simulink model "FOC_Motor_Sensorless"  (R2025b)
settings: Solver=VariableStepAuto  StartTime=0.0  StopTime=8  RelTol=1e-3
undefined symbols (not defined in the file or in its folder): adc, dataRange, encoder, inverter, paramAdcAmperePerCount, paramAdcCalibrationSamples, paramAdcCountAtZeroAmpere, paramAdcEnablecalibration, paramCurrentControlSatVoltage, paramOverCurrentDuration, paramOverCurrentEnable, paramOverCurrentLimit, paramPwmCompareAtZeroVolt, paramPwmCompareMax, paramPwmComparePerVolt, paramVelocityControlSatCurrent, PI_params, pmsm, PU_System, pwm, sampleTime
libraries: fl_lib x12, nesl_utility x12, mcbeeMathTransformLib x5, mcbcontrolslib x5, ee_lib x4, slpidlib x2, simulink x2, mcbhdlpositiondecoderlib x2, mcbplantlib x1, autolibpmsmexterior x1, eeGeneralControl x1, SignalEditorBlockLib x1
(part 2 of 2)

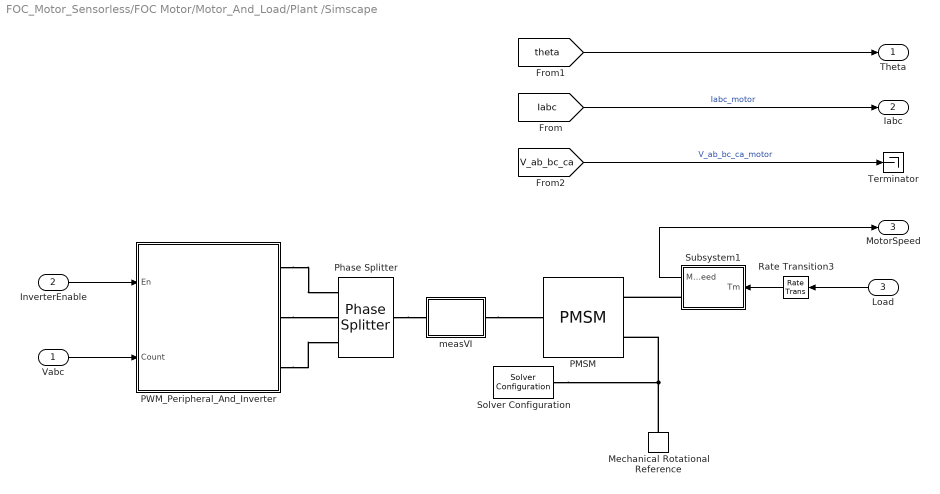
== system FOC_Motor_Sensorless/FOC Motor/Motor_And_Load/Plant /Simscape ==
  Vabc : Inport
  InverterEnable : Inport  Port=2
  Load : Inport  Port=3
  Mechanical Rotational Reference : fl_lib/Mechanical/Rotational Elements/Mechanical Rotational Reference
  PMSM : ee_lib/Electromechanical/Permanent Magnet/PMSM  port_option=ee.enum.threePhasePort.composite  winding_type=ee.enum.statorconnection.wye  machine_param=ee.enum.pmsm.parameterization.constant  nPolePairs=pmsm.p  pmflux_param=ee.enum.pmflux.fluxlinkage  pm_flux_linkage=pmsm.FluxPM Wb  torque_constant=0.18 N*m/A  back_emf_constant=0.18 V/(rad/s)  stator_param=ee.enum.statorparam.LdLqL0  Ld=pmsm.Ld H  Lq=pmsm.Lq H  idVec=[-200, 0, 200] A  iqVec=[-200, 0, 200] A  LdMatrix=0.0002 * ones(3, 3) H  LqMatrix=0.0002 * ones(3, 3) H  PmMatrix=0.1 * ones(3, 3) Wb  ktMatrix=0.18 * ones(3, 3) N*m/A  keMatrix=0.18 * ones(3, 3) V/(rad/s)  L0=0 H  Ls=0.0002 H  Lm=-0.00002 H  Ms=0.00002 H  Rs=pmsm.Rs Ohm  zero_sequence=ee.enum.park.zerosequence.exclude  axes_param=ee.enum.rotorangle.daxis  loss_param=ee.enum.ironloss.none  losses_oc=[0, 0, 0] W  losses_sc=[0, 0, 0] W  f_losses=60 Hz  Isc_losses=95 A  J=pmsm.J kg*m^2  lam=pmsm.B N*m/(rad/s)  i_d_specify=off  i_d_priority=None  i_d=0 A  i_d_nominal_specify=off  i_d_nominal_value=1  i_d_nominal_unit=A  i_q_specify=off  i_q_priority=None  i_q=0 A  i_q_nominal_specify=off  i_q_nominal_value=1  i_q_nominal_unit=A  torque_specify=off  torque_priority=None  torque=0 N*m  torque_nominal_specify=off  torque_nominal_value=1  torque_nominal_unit=N*m  angular_velocity_specify=off  angular_velocity_priority=High  angular_velocity=0 rpm  angular_velocity_nominal_specify=off  angular_velocity_nominal_value=1  angular_velocity_nominal_unit=rpm  angular_position_specify=off  angular_position_priority=High  angular_position=0 deg  angular_position_nominal_specify=off  angular_position_nominal_value=1  angular_position_nominal_unit=deg  alpha=3.93e-3 1/K  alpha_flux=-0.001 1/K  Tmeas=298.15 K  stator_thermal_mass=100 J/K  rotor_thermal_mass=200 J/K  Rm_percent_rotor=90  Rd_percent_rotor=30  temperatureA_specify=off  temperatureA_priority=High  temperatureA=25 degC  temperatureA_nominal_specify=off  temperatureA_nominal_value=1  temperatureA_nominal_unit=degC  temperatureB_specify=off  temperatureB_priority=High  temperatureB=25 degC  temperatureB_nominal_specify=off  temperatureB_nominal_value=1  temperatureB_nominal_unit=degC  temperatureC_specify=off  temperatureC_priority=High  temperatureC=25 degC  temperatureC_nominal_specify=off  temperatureC_nominal_value=1  temperatureC_nominal_unit=degC  temperatureR_specify=off  temperatureR_priority=High  temperatureR=25 degC  temperatureR_nominal_specify=off  temperatureR_nominal_value=1  temperatureR_nominal_unit=degC
      settings: InternalSimscapePortConfiguration="{\"Bottom\":[],\"Left\":[{\"id\":\"N\",\"label\":\"~\",\"type\":\"foundation.electrical.three_phase\"}],\"Right\":[{\"id\":\"R\",\"label\":\"R\",\"type\":\"foundation.mechanical.rotational.rotational\"},{\"id\":\"C\",\"label\":\"C\",\"type\":\"foundation.mechanical.rotational.rotational\"}],\"Top\":[]}"
  PWM_Peripheral_And_Inverter : Subsystem  VariantControl=variantPwm == enumPwm.behavior
      mask Display:
      | image('pwmPeripheralAndInverterMask.png')
      | port_label('input',1,'En')
      | port_label('input',2,'Compare')
      | text(0.98, 0.64, 'A', 'HorizontalAlignment', 'Right')
      | text(0.98, 0.38, 'B', 'HorizontalAlignment', 'Right')
      | text(0.98, 0.12, 'C', 'HorizontalAlignment', 'Right')
  Phase Splitter : ee_lib/Connectors & References/Phase Splitter
  Rate Transition3 : RateTransition  Deterministic=off  OutPortSampleTime=sampleTime.CurrentControl/2
  Solver Configuration : nesl_utility/Solver Configuration  PhysicalDomain=network_engine_domain  SubClassName=solver  LeftPortType=input  RightPortType=generic  Tones=[]  Harmonics=[]  SimulateNoise=off  Profile=off  UseLocalSampling=off  EnableSwitchedLinearOptims=on  FrequencyDomain=off  UseCCode=off  RelTol=0.001  AbsTol=1e-06  MinStep=1e-09  ToWorkspace=off  RevertToSquareIcSolve=off  NumHomotopyIterations=100  PhasorMode=off  PhasorModeNumHarmonics=1  ConsistencySolver=NEWTON_FTOL  IndexReductionMethod=DerivativeReplacement  DoDC=off  ResidualTolerance=1e-09  ConsistencyTolSource=GLOBAL  ConsistencyAbsTol=0.001  ConsistencyRelTol=0.001  ConsistencyTolFactor=0.001  UseLocalSolver=on  LocalSolverChoice=NE_BACKWARD_EULER_ADVANCER  ResolveIndetEquations=on  FunctionEvalNumThread=1  LocalSolverSampleTime=sampleTime.CurrentControl/2  DoFixedCost=on  MaxNonlinIter=3  MaxModeIter=2  ComputeImpulses=off  ImpulseIterations=1  LinearAlgebra=Full  LinearAlgebraNumThread=0  EquationFormulation=NE_TIME_EF  DelaysMemoryBudget=1024  AutomaticFiltering=off  FilteringTimeConstant=0.001  PartitionStorageMethod=AS_NEEDED  PartitionMemoryBudget=1024  PartitionMethod=ROBUST  MultibodyUseLocalSolver=off  MultibodyLocalSolverChoice=ODE1  MultibodyLocalSolverSampleTime=0.001
  Subsystem1 : Subsystem
  Terminator : Terminator
  measVI : Subsystem
  Theta : Outport
  Iabc : Outport  Port=2
  MotorSpeed : Outport  Port=3
  wires:
  Subsystem1/1(MotorSpeed) -> MotorSpeed/1
  [V_ab_bc_ca] -> Terminator/1  "V_ab_bc_ca_motor"
  Rate Transition3/1 -> Subsystem1/1(Tm)
  [theta] -> Theta/1
  [Iabc] -> Iabc/1  "Iabc_motor"
  Load/1 -> Rate Transition3/1
  Vabc/1 -> PWM_Peripheral_And_Inverter/2(Count)
  InverterEnable/1 -> PWM_Peripheral_And_Inverter/1(En)
  connections:
  Subsystem1/RConn1 -- PMSM/RConn1
  Mechanical Rotational Reference/LConn1 -- PMSM/RConn2 -- Solver Configuration/RConn1
  measVI/RConn1 -- PMSM/LConn1
  Phase Splitter/LConn1 -- measVI/LConn1
  PWM_Peripheral_And_Inverter/RConn1 -- Phase Splitter/RConn1
  PWM_Peripheral_And_Inverter/RConn2 -- Phase Splitter/RConn2
  PWM_Peripheral_And_Inverter/RConn3 -- Phase Splitter/RConn3

== system FOC_Motor_Sensorless/FOC Motor/Motor_And_Load/Sensor_Measurements/Get_PU  ==
  rad : Inport
  Constant2 : Constant  Value=2*pi  OutDataTypeStr=single  SampleTime=-1
  Get_PU : Gain  Gain=1/(2*pi)  RndMeth=Simplest  OutDataTypeStr=Inherit: Same as input
  Mod : Math  Operator=mod
  PU : Outport  VectorParamsAs1DForOutWhenUnconnected=off
  wires:
  rad/1 -> Mod/1
  Constant2/1 -> Mod/2
  Mod/1 -> Get_PU/1
  Get_PU/1 -> PU/1

== system FOC_Motor_Sensorless/FOC Motor/Motor_And_Load/Sensor_Measurements/Wrap ==
  in : Inport
  Constant2 : Constant  OutDataTypeStr=single  SampleTime=-1
  Mod : Math  Operator=mod
  out : Outport  VectorParamsAs1DForOutWhenUnconnected=off
  wires:
  in/1 -> Mod/1
  Constant2/1 -> Mod/2
  Mod/1 -> out/1

== system FOC_Motor_Sensorless/FOC Motor/Controller_Algorithm_Local/Algorithm_HDL/FOC_Current_Control/ADC_Count_To_Current ==
  note: ADC Count to Current
  Count : Inport  OutMin=0  OutMax=2^16-1  OutDataTypeStr=uint16  LockScale=on
  ADC_Offsets : Inport  Port=2
  Add : Sum  Inputs=+-  OutDataTypeStr=int16  LockScale=on
  Data_Type_Convert : DataTypeConversion  OutDataTypeStr=int32  SaturateOnIntegerOverflow=off  RndMeth=Floor  LockScale=on
  Product : Product  OutDataTypeStr=fixdt(1,32,19)
  Sat : Saturate  UpperLimit=dataRange.PhaseCurrent.Max  LowerLimit=dataRange.PhaseCurrent.Min  OutDataTypeStr=fixdt(1,16,11)
      settings: AttributesFormatString=-----------------\nLower = %<LowerLimit>\nUpper = %<UpperLimit>
  Scalar : Constant  Value=paramAdcAmperePerCount  OutDataTypeStr=fixdt(1,16,19)  SampleTime=-1
  Current : Outport  VectorParamsAs1DForOutWhenUnconnected=off
  ADC_Counts : Outport  Port=2  VectorParamsAs1DForOutWhenUnconnected=off
  wires:
  ADC_Offsets/1 -> Add/2
  Scalar/1 -> Product/2
  Add/1 -> Product/1
  Count/1 -> ADC_Counts/1, Data_Type_Convert/1
  Data_Type_Convert/1 -> Add/1
  Product/1 -> Sat/1
  Sat/1 -> Current/1

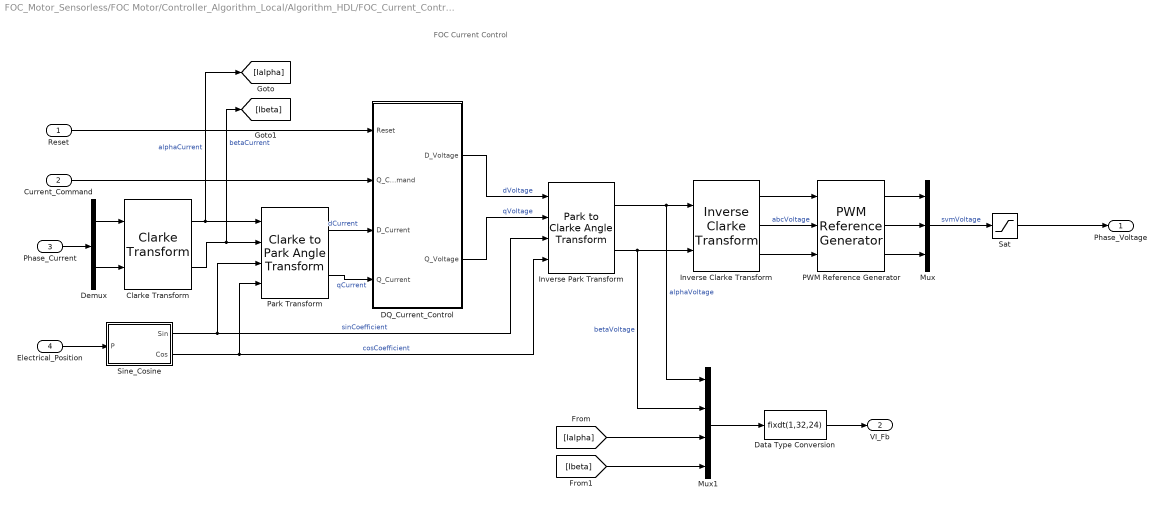
== system FOC_Motor_Sensorless/FOC Motor/Controller_Algorithm_Local/Algorithm_HDL/FOC_Current_Control/FOC_Current_Control ==
  note: FOC Current Control
  Reset : Inport  SampleTime=sampleTime.CurrentControl
  Current_Command : Inport  Port=2  OutMin=dataRange.PhaseCurrent.Min  OutMax=dataRange.PhaseCurrent.Max  OutDataTypeStr=fixdt(1,16,11)  SampleTime=sampleTime.CurrentControl
  Phase_Current : Inport  Port=3  OutMin=dataRange.PhaseCurrent.Min  OutMax=dataRange.PhaseCurrent.Max  OutDataTypeStr=fixdt(1,16,11)  SampleTime=sampleTime.CurrentControl
  Electrical_Position : Inport  Port=4  OutMin=0  OutMax=2*pi  OutDataTypeStr=fixdt(1,16,12)  SampleTime=sampleTime.CurrentControl
  Clarke Transform : mcbeeMathTransformLib/Clarke Transform  VariantControl=Variant2  PowerInvariant=off  UseWithEmbedded=on  PhaseInput=Two inputs
      settings: LibrarySourceBlock=mcbcontrolslib/Clarke Transform
  DQ_Current_Control : Subsystem
  Data Type Conversion : DataTypeConversion  OutDataTypeStr=fixdt(1,32,24)  SaturateOnIntegerOverflow=off  RndMeth=Floor
  Demux : Demux  Outputs=2
  Inverse Clarke Transform : mcbeeMathTransformLib/Inverse Clarke Transform  PowerInvariant=off  UseWithEmbedded=on  PhaseInput=Two inputs
      settings: LibrarySourceBlock=mcbcontrolslib/Inverse Clarke Transform
  Inverse Park Transform : mcbeeMathTransformLib/Park to Clarke Angle Transform  AxisAlignment=D-axis  UseWithEmbedded=on  PhaseInput=Two inputs  ThetaInput=Sine and Cosine electrical position  AngleInput=Per-unit  N_points=1024
      settings: LibrarySourceBlock=mcbcontrolslib/Inverse Park Transform
  Mux : Mux  Inputs=3
  Mux1 : Mux
  PWM Reference Generator : mcbcontrolslib/PWM Reference Generator  inSignal=Vabc  modType=SVM: space vector modulation
      settings: LibrarySourceBlock=mcbhdllib/Controls/Math Transforms/PWM Reference Generator
  Park Transform : mcbeeMathTransformLib/Clarke to Park Angle Transform  AxisAlignment=D-axis  UseWithEmbedded=on  PhaseInput=Two inputs  ThetaInput=Sine and Cosine electrical position  AngleInput=Per-unit  N_points=1024
      settings: LibrarySourceBlock=mcbcontrolslib/Park Transform
  Sat : Saturate  UpperLimit=dataRange.PhaseVoltage.Max  LowerLimit=dataRange.PhaseVoltage.Min  OutDataTypeStr=fixdt(1,16,11)
      settings: AttributesFormatString=-----------------\nLower = %<LowerLimit>\nUpper = %<UpperLimit>
  Sine_Cosine : Subsystem
  Phase_Voltage : Outport  SampleTime=sampleTime.CurrentControl  VectorParamsAs1DForOutWhenUnconnected=off
  VI_Fb : Outport  Port=2
  wires:
  Sine_Cosine/1(Sin) -> Inverse Park Transform/3, Park Transform/3  "sinCoefficient"
  Sine_Cosine/2(Cos) -> Park Transform/4, Inverse Park Transform/4  "cosCoefficient"
  Electrical_Position/1 -> Sine_Cosine/1(P)
  Phase_Current/1 -> Demux/1
  Clarke Transform/1 -> [Ialpha], Park Transform/1  "alphaCurrent"
  Clarke Transform/2 -> [Ibeta], Park Transform/2  "betaCurrent"
  Inverse Park Transform/1 -> Mux1/1, Inverse Clarke Transform/1  "alphaVoltage"
  Inverse Park Transform/2 -> Mux1/2, Inverse Clarke Transform/2  "betaVoltage"
  Park Transform/1 -> DQ_Current_Control/3(D_Current)  "dCurrent"
  Park Transform/2 -> DQ_Current_Control/4(Q_Current)  "qCurrent"
  Current_Command/1 -> DQ_Current_Control/2(Q_Command)
  DQ_Current_Control/1(D_Voltage) -> Inverse Park Transform/1  "dVoltage"
  DQ_Current_Control/2(Q_Voltage) -> Inverse Park Transform/2  "qVoltage"
  Mux/1 -> Sat/1  "svmVoltage"
  Sat/1 -> Phase_Voltage/1
  Reset/1 -> DQ_Current_Control/1(Reset)
  Demux/1 -> Clarke Transform/1
  Demux/2 -> Clarke Transform/2
  Inverse Clarke Transform/1 -> PWM Reference Generator/1
  Inverse Clarke Transform/2 -> PWM Reference Generator/2  "abcVoltage"
  Inverse Clarke Transform/3 -> PWM Reference Generator/3
  PWM Reference Generator/1 -> Mux/1
  PWM Reference Generator/2 -> Mux/2
  PWM Reference Generator/3 -> Mux/3
  Mux1/1 -> Data Type Conversion/1
  Data Type Conversion/1 -> VI_Fb/1
  [Ibeta] -> Mux1/4
  [Ialpha] -> Mux1/3

== system FOC_Motor_Sensorless/FOC Motor/Controller_Algorithm_Local/Algorithm_HDL/FOC_Current_Control/FO_Position_Velocity ==
  note: Fo Position And Velocity
  VIFb : Inport
  Reset : Inport  Port=2
  Data Type Conversion : DataTypeConversion  OutDataTypeStr=fixdt(1,16,12)  SaturateOnIntegerOverflow=off  RndMeth=Floor
  Data Type Conversion1 : DataTypeConversion  SaturateOnIntegerOverflow=off  RndMeth=Floor
  Data Type Conversion2 : DataTypeConversion  OutDataTypeStr=fixdt(1,16,5)  SaturateOnIntegerOverflow=off  RndMeth=Floor
  Demux : Demux
  Flux Observer : mcbhdlpositiondecoderlib/Flux Observer  DataTypeSelect=off  ParameterBusInput=off  MotorSelection=PMSM  BlockInputUnit=SI unit  PerUnitVoltage=13.86  PerUnitCurrent=19.3  PositionSelect=on  FluxSelect=off  TorqueSelect=off  PolePairs=4  StatorResistance=pmsm.Rs  StatorDAxisInductance=pmsm.Ld  StatorLeakageInductance=0.0068  RotorLeakageInductance=0.0068  MagnetizingInductance=0.0300  CutoffFreq=3.1863  BlockSampleTime=sampleTime.CurrentControl  PositionUnit=Radians  PositionDatatype=fixdt(1,32,24)  FluxUnit=Weber  PerUnitFlux=0.1  FluxDatatype=fixdt(1,16,11)  TorqueUnit=Nm  PerUnitTorque=100  TorqueDatatype=fixdt(1,16,11)  DataType=0
      settings: LibrarySourceBlock=mcbhdllib/Sensorless Estimators/Flux Observer
  NOT : Logic  Operator=NOT  IconShape=distinctive  AllPortsSameDT=off  OutDataTypeStr=boolean
  Speed Measurement1 : mcbhdlpositiondecoderlib/Speed Measurement  PositionUnit=Radians  PositionScalingDatatype=uint32  SpeedCalculationMode=Time interval for speed calculation  SampleTimeAsync=sampleTime.EncoderPosition  MaximumApplicationSpeed=1000  SpeedResolution=5e-6  DelayLength=30  MaximumMeasurableSpeed=24999  MeasurableSpeedResolution=1.1642e-05  SpeedUnit=Radians/Sec  PerUnitSpeed=1000  SpeedDataType=fixdt(1,32,18)
      settings: LibrarySourceBlock=mcbhdllib/Sensor Decoders/Speed Measurement
  elect2mech : Gain  Gain=1/pmsm.p  RndMeth=Simplest  OutDataTypeStr=Inherit: Same as input
  Rotor_Position : Outport  VectorParamsAs1DForOutWhenUnconnected=off
  Electrical_Position : Outport  Port=2  VectorParamsAs1DForOutWhenUnconnected=off
  Rotor_Velocity : Outport  Port=3  VectorParamsAs1DForOutWhenUnconnected=off
  wires:
  Speed Measurement1/1 -> elect2mech/1
  Flux Observer/1 -> Speed Measurement1/1, Data Type Conversion1/1
  elect2mech/1 -> Data Type Conversion2/1
  Demux/1 -> Flux Observer/1
  Demux/2 -> Flux Observer/2
  Demux/3 -> Flux Observer/3
  Demux/4 -> Flux Observer/4
  Reset/1 -> NOT/1
  NOT/1 -> Flux Observer/5
  Data Type Conversion/1 -> Rotor_Position/1
  VIFb/1 -> Demux/1
  Data Type Conversion1/1 -> Data Type Conversion/1, Electrical_Position/1
  Data Type Conversion2/1 -> Rotor_Velocity/1

== system FOC_Motor_Sensorless/FOC Motor/Controller_Algorithm_Local/Algorithm_HDL/FOC_Current_Control/Over_Current_Detector ==
  note: Over Current Detector
  Motor_On : Inport  OutMin=0  OutMax=1  OutDataTypeStr=boolean  LockScale=on
  Phase_Current : Inport  Port=2  OutMin=dataRange.PhaseCurrent.Min  OutMax=dataRange.PhaseCurrent.Max  OutDataTypeStr=fixdt(1,16,11)
  AND : Logic  IconShape=distinctive  AllPortsSameDT=off  OutDataTypeStr=boolean
  AND1 : Logic  IconShape=distinctive  AllPortsSameDT=off  OutDataTypeStr=boolean
  Abs : Abs  SaturateOnIntegerOverflow=off
      settings: LockScale=on
  Demux : Demux  Outputs=2
  Detect_Over_Current_Error : Stateflow chart  TreatAsAtomicUnit=on
  Enable_Over_Current_Detection : Constant  Value=paramOverCurrentEnable  OutDataTypeStr=boolean  SampleTime=-1  LockScale=on
  Motor_On1 : InportShadow  OutMin=0  OutMax=1  OutDataTypeStr=boolean
      settings: LockScale=on
  NOT : Logic  Operator=NOT  IconShape=distinctive  AllPortsSameDT=off  OutDataTypeStr=boolean
  Over_Current_Duration : Constant  Value=paramOverCurrentDuration  OutDataTypeStr=fixdt(1,16,14)  SampleTime=-1
  Over_Current_Limit : Constant  Value=paramOverCurrentLimit  OutDataTypeStr=fixdt(1,16,11)  SampleTime=-1
  Tick_Per_Sec : Gain  Gain=1/sampleTime.OverCurrentDetector  ParamDataTypeStr=fixdt(1,16,0)  OutDataTypeStr=uint16  LockScale=on
      settings: AttributesFormatString=---------------------------\nGain = %<Gain>
  En_Inv : Outport  VectorParamsAs1DForOutWhenUnconnected=off
  Error : Outport  Port=2  VectorParamsAs1DForOutWhenUnconnected=off
  wires:
  Tick_Per_Sec/1 -> Detect_Over_Current_Error/5(overCurrentDurationTicks)
  Phase_Current/1 -> Abs/1
  Abs/1 -> Demux/1
  Demux/2 -> Detect_Over_Current_Error/3(phaseCurrentB)
  Detect_Over_Current_Error/1(error) -> Error/1, NOT/1  "overCurrentErrorDetected"
  Over_Current_Duration/1 -> Tick_Per_Sec/1
  Over_Current_Limit/1 -> Detect_Over_Current_Error/4(overCurrentLimit)
  Demux/1 -> Detect_Over_Current_Error/2(phaseCurrentA)
  Motor_On/1 -> AND/1
  AND1/1 -> En_Inv/1  "enableInverter"
  NOT/1 -> AND1/2
  Motor_On1/1 -> AND1/1
  AND/1 -> Detect_Over_Current_Error/1(enableOverCurrentDetect)
  Enable_Over_Current_Detection/1 -> AND/2

== system FOC_Motor_Sensorless/FOC Motor/Controller_Algorithm_Local/Algorithm_HDL/FOC_Current_Control/Voltage_To_PWM_Compare ==
  note: Voltage To PWM Compare
  Voltage : Inport  OutMin=dataRange.PhaseVoltage.Min  OutMax=dataRange.PhaseVoltage.Max  OutDataTypeStr=fixdt(1,16,11)
  Add : Sum  OutDataTypeStr=fixdt(1,32,17)
  Bias : Constant  Value=paramPwmCompareAtZeroVolt  OutDataTypeStr=fixdt(1,16,2)  SampleTime=-1
  Data_Type_Conversion : DataTypeConversion  OutDataTypeStr=uint16  SaturateOnIntegerOverflow=off  RndMeth=Floor  LockScale=on
  Saturation : Saturate  UpperLimit=paramPwmCompareMax  LowerLimit=0
      settings: AttributesFormatString=|
      | --------------------------------
      | Upper Limit = %<UpperLimit>
      | Lower Limit = %<LowerLimit>
  Slope : Gain  Gain=paramPwmComparePerVolt  ParamDataTypeStr=fixdt(1,16,6)  OutDataTypeStr=fixdt(1,32,18)
      settings: AttributesFormatString=|
      | ----------------------------------------
      | Gain = %<Gain>
  Compare : Outport  VectorParamsAs1DForOutWhenUnconnected=off
  wires:
  Data_Type_Conversion/1 -> Compare/1  "pwmCompare"
  Voltage/1 -> Slope/1  "phaseVoltage"
  Slope/1 -> Add/1
  Saturation/1 -> Data_Type_Conversion/1
  Bias/1 -> Add/2
  Add/1 -> Saturation/1

== system FOC_Motor_Sensorless/FOC Motor/Controller_Algorithm_Local/Algotithm_C/Open_Loop_Velocity_Control/Open_Loop_Control ==
  OpenLoopSpeed : Inport
  Gain : Gain  Gain=sampleTime.VelocityControl*PU_System.N_base*pmsm.p/60  OutDataTypeStr=Inherit: Same as input  ParamDataTypeStr=Inherit: Same as input
  Position Generator : mcbcontrolslib/Position Generator  AngleOutput=Per-unit  InitialThetaSource=Specify via dialog  ExternalReset=none  Offset=0
  Pos_PU_Out : Outport
  wires:
  Position Generator/1 -> Pos_PU_Out/1
  Gain/1 -> Position Generator/1
  OpenLoopSpeed/1 -> Gain/1

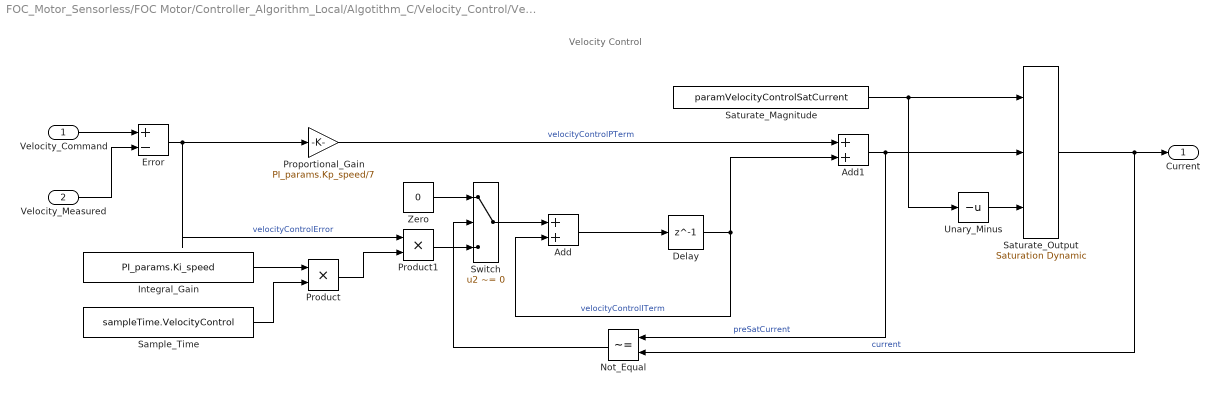
== system FOC_Motor_Sensorless/FOC Motor/Controller_Algorithm_Local/Algotithm_C/Velocity_Control/Velocity_Control ==
  note: Velocity Control
  Velocity_Command : Inport  SampleTime=sampleTime.VelocityControl
  Velocity_Measured : Inport  Port=2  SampleTime=sampleTime.VelocityControl
  Add : Sum
  Add1 : Sum
  Delay : Delay  DelayLength=1
  Error : Sum  Inputs=+-
  Integral_Gain : Constant  Value=PI_params.Ki_speed  OutDataTypeStr=Inherit: Inherit via back propagation
  Not_Equal : RelationalOperator  Operator=~=  OutDataTypeStr=boolean  InputSameDT=off
  Product : Product  OutDataTypeStr=Inherit: Same as first input
  Product1 : Product  OutDataTypeStr=Inherit: Same as first input
  Proportional_Gain : Gain  Gain=PI_params.Kp_speed/7
      settings: AttributesFormatString=|
      | -----------------------------------
      | Gain = %<Gain>
  Sample_Time : Constant  Value=sampleTime.VelocityControl  OutDataTypeStr=Inherit: Inherit via back propagation
  Saturate_Magnitude : Constant  Value=paramVelocityControlSatCurrent  OutDataTypeStr=Inherit: Inherit via back propagation
  Saturate_Output : simulink/Discontinuities/Saturation Dynamic  OutMin=[]  OutMax=[]  OutDataTypeStr=Inherit: Same as second input  OutDataType=fixdt(1, 16)  OutScaling=2^-10  DoSatur=off
  Switch : Switch  Criteria=u2 ~= 0  SaturateOnIntegerOverflow=off  InputSameDT=off
  Unary_Minus : UnaryMinus
  Zero : Constant  Value=0  OutDataTypeStr=Inherit: Inherit via back propagation
  Current : Outport  SampleTime=sampleTime.VelocityControl  VectorParamsAs1DForOutWhenUnconnected=off
  wires:
  Add/1 -> Delay/1
  Product1/1 -> Switch/3
  Product/1 -> Product1/2
  Sample_Time/1 -> Product/2
  Integral_Gain/1 -> Product/1
  Unary_Minus/1 -> Saturate_Output/3
  Saturate_Magnitude/1 -> Unary_Minus/1, Saturate_Output/1
  Zero/1 -> Switch/1
  Switch/1 -> Add/1
  Not_Equal/1 -> Switch/2
  Saturate_Output/1 -> Not_Equal/2, Current/1  "current"
  Error/1 -> Product1/1, Proportional_Gain/1  "velocityControlError"
  Proportional_Gain/1 -> Add1/1  "velocityControlPTerm"
  Velocity_Command/1 -> Error/1
  Add1/1 -> Saturate_Output/2, Not_Equal/1  "preSatCurrent"
  Delay/1 -> Add1/2, Add/2  "velocityControlITerm"
  Velocity_Measured/1 -> Error/2

== system FOC_Motor_Sensorless/FOC Motor/Motor_And_Load/Plant /MCB/Inverter ==
  note: Inverter
  Duty : Inport
  Average-Value Inverter : mcbplantlib/Average-Value Inverter
  Constant2 : Constant  Value=inverter.V_dc  OutDataTypeStr=single  SampleTime=-1
  Data Type Conversion1 : DataTypeConversion  OutDataTypeStr=single  RndMeth=Simplest  SaturateOnIntegerOverflow=off
  Rate Transition3 : RateTransition  Deterministic=off  OutPortSampleTime=sampleTime.CurrentControl/2
  Vabc_motor : Outport
  wires:
  Constant2/1 -> Average-Value Inverter/2
  Rate Transition3/1 -> Average-Value Inverter/1
  Duty/1 -> Data Type Conversion1/1
  Average-Value Inverter/1 -> Vabc_motor/1  "Vabc_motor"
  Data Type Conversion1/1 -> Rate Transition3/1

== system FOC_Motor_Sensorless/FOC Motor/Motor_And_Load/Plant /MCB/PWM_Count_to_Duty ==
  <pwmCompare> : Inport
  Add : Sum  Inputs=+-
  Bias : Constant  Value=paramPwmCompareAtZeroVolt  OutDataTypeStr=single  SampleTime=-1
  Constant : Constant  Value=0.5  OutDataTypeStr=single  SampleTime=-1
  Data Type Conversion : DataTypeConversion  OutDataTypeStr=single  SaturateOnIntegerOverflow=off  RndMeth=Floor
  Normalize [-0.5 to 0.5] : Gain  Gain=1/ (2 * inverter.V_dc / sqrt(3))  OutDataTypeStr=single  RndMeth=Simplest
  Slope : Gain  Gain=1/paramPwmComparePerVolt  ParamDataTypeStr=fixdt(1,16,6)  OutDataTypeStr=single
      settings: AttributesFormatString=|
      | ----------------------------------------
      | Gain = %<Gain>
  Sum : Sum  Inputs=|++
  Duty : Outport
  wires:
  Constant/1 -> Sum/2
  Normalize [-0.5 to 0.5]/1 -> Sum/1
  <pwmCompare>/1 -> Data Type Conversion/1
  Sum/1 -> Duty/1
  Data Type Conversion/1 -> Add/1
  Bias/1 -> Add/2
  Add/1 -> Slope/1
  Slope/1 -> Normalize [-0.5 to 0.5]/1

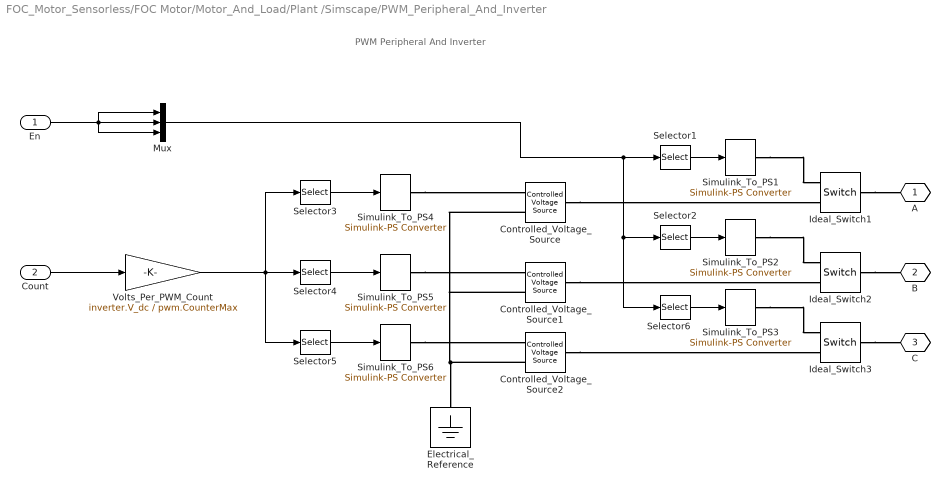
== system FOC_Motor_Sensorless/FOC Motor/Motor_And_Load/Plant /Simscape/PWM_Peripheral_And_Inverter ==
  note: PWM Peripheral And Inverter
  En : Inport
  Count : Inport  Port=2
  Controlled_Voltage_Source : fl_lib/Electrical/Electrical Sources/Controlled Voltage Source
  Controlled_Voltage_Source1 : fl_lib/Electrical/Electrical Sources/Controlled Voltage Source
  Controlled_Voltage_Source2 : fl_lib/Electrical/Electrical Sources/Controlled Voltage Source
  Electrical_Reference : fl_lib/Electrical/Electrical Elements/Electrical Reference
  Ideal_Switch1 : fl_lib/Electrical/Electrical Elements/Switch  R_closed=0.0001 Ohm  G_open=1e-5 1/Ohm  Threshold=0  i_specify=off  i_priority=None  i=0 A  i_nominal_specify=off  i_nominal_value=1  i_nominal_unit=A  v_specify=off  v_priority=None  v=0 V  v_nominal_specify=off  v_nominal_value=1  v_nominal_unit=V
  Ideal_Switch2 : fl_lib/Electrical/Electrical Elements/Switch  R_closed=0.0001 Ohm  G_open=1e-5 1/Ohm  Threshold=0  i_specify=off  i_priority=None  i=0 A  i_nominal_specify=off  i_nominal_value=1  i_nominal_unit=A  v_specify=off  v_priority=None  v=0 V  v_nominal_specify=off  v_nominal_value=1  v_nominal_unit=V
  Ideal_Switch3 : fl_lib/Electrical/Electrical Elements/Switch  R_closed=0.0001 Ohm  G_open=1e-5 1/Ohm  Threshold=0  i_specify=off  i_priority=None  i=0 A  i_nominal_specify=off  i_nominal_value=1  i_nominal_unit=A  v_specify=off  v_priority=None  v=0 V  v_nominal_specify=off  v_nominal_value=1  v_nominal_unit=V
  Mux : Mux  Inputs=3
  Selector1 : Selector  InputPortWidth=3  IndexOptions=Index vector (dialog)  Indices=[1]  OutputSizes=1
  Selector2 : Selector  InputPortWidth=3  IndexOptions=Index vector (dialog)  Indices=2  OutputSizes=1
  Selector3 : Selector  InputPortWidth=3  IndexOptions=Index vector (dialog)  Indices=[1]  OutputSizes=1
  Selector4 : Selector  InputPortWidth=3  IndexOptions=Index vector (dialog)  Indices=2  OutputSizes=1
  Selector5 : Selector  InputPortWidth=3  IndexOptions=Index vector (dialog)  Indices=3  OutputSizes=1
  Selector6 : Selector  InputPortWidth=3  IndexOptions=Index vector (dialog)  Indices=3  OutputSizes=1
  Simulink_To_PS{1..6} (6 alike) : nesl_utility/Simulink-PS Converter  PhysicalDomain=network_engine_domain  SubClassName=ps_input  LeftPortType=input  RightPortType=output  PseudoPeriodic=off  Frequencies=[]  NoiseDistribution=none  NoiseParameters=[]  Unit=1  AffineConversion=off  FilteringAndDerivatives=zero  SimscapeFilterOrder=1  InputFilterTimeConstant=0.001  UdotUserProvided=1
  Volts_Per_PWM_Count : Gain  Gain=inverter.V_dc / pwm.CounterMax  ParamDataTypeStr=double  OutDataTypeStr=double
      settings: AttributesFormatString=|
      | ----------------------------------------------------------------
      | Gain = %<Gain>
  A : PMIOPort  Tag=PMCPort  Side=Right
  B : PMIOPort  Tag=PMCPort  Port=2  Side=Right
  C : PMIOPort  Tag=PMCPort  Port=3  Side=Right
  wires:
  Selector1/1 -> Simulink_To_PS1/1
  Selector3/1 -> Simulink_To_PS4/1
  Selector4/1 -> Simulink_To_PS5/1
  Selector5/1 -> Simulink_To_PS6/1
  Volts_Per_PWM_Count/1 -> Selector5/1, Selector3/1, Selector4/1
  Count/1 -> Volts_Per_PWM_Count/1
  Selector2/1 -> Simulink_To_PS2/1
  Selector6/1 -> Simulink_To_PS3/1
  En/1 -> Mux/3, Mux/2, Mux/1
  Mux/1 -> Selector6/1, Selector2/1, Selector1/1
  connections:
  Ideal_Switch1/LConn1 -- A/RConn1
  Ideal_Switch2/LConn1 -- B/RConn1
  Ideal_Switch3/LConn1 -- C/RConn1
  Simulink_To_PS1/RConn1 -- Ideal_Switch1/RConn1
  Simulink_To_PS2/RConn1 -- Ideal_Switch2/RConn1
  Simulink_To_PS3/RConn1 -- Ideal_Switch3/RConn1
  Simulink_To_PS4/RConn1 -- Controlled_Voltage_Source/RConn1
  Controlled_Voltage_Source/LConn1 -- Ideal_Switch1/RConn2
  Controlled_Voltage_Source1/LConn1 -- Ideal_Switch2/RConn2
  Controlled_Voltage_Source2/LConn1 -- Ideal_Switch3/RConn2
  Simulink_To_PS6/RConn1 -- Controlled_Voltage_Source2/RConn1
  Simulink_To_PS5/RConn1 -- Controlled_Voltage_Source1/RConn1
  Controlled_Voltage_Source2/RConn2 -- Controlled_Voltage_Source/RConn2 -- Controlled_Voltage_Source1/RConn2 -- Electrical_Reference/LConn1

== system FOC_Motor_Sensorless/FOC Motor/Motor_And_Load/Plant /Simscape/Subsystem1 ==
  Tm : Inport
  Data Type Conversion1 : DataTypeConversion  SaturateOnIntegerOverflow=off  RndMeth=Floor
  Gain : Gain  Gain=2*pi/60
  Gain1 : Gain  Gain=-1
  Ideal Rotational Motion Sensor : fl_lib/Mechanical/Mechanical Sensors/Ideal Rotational Motion Sensor  reference=foundation.enum.MeasurementReference.difference  acceleration_port=false  velocity_port=true  position_port=true  wrap_angle=simscape.enum.onoff.off  offset=0 rad
  Ideal Torque Source : fl_lib/Mechanical/Mechanical Sources/Ideal Torque Source
  Mechanical Rotational Reference1 : fl_lib/Mechanical/Rotational Elements/Mechanical Rotational Reference
  Mechanical Rotational Reference2 : fl_lib/Mechanical/Rotational Elements/Mechanical Rotational Reference
  PS-Simulink Converter : nesl_utility/PS-Simulink Converter  PhysicalDomain=network_engine_domain  SubClassName=ps_output  LeftPortType=input  RightPortType=output  PseudoPeriodic=off  Frequencies=[]  VectorFormat=1-D array  Unit=rpm  AffineConversion=off
  PS-Simulink Converter1 : nesl_utility/PS-Simulink Converter  PhysicalDomain=network_engine_domain  SubClassName=ps_output  LeftPortType=input  RightPortType=output  PseudoPeriodic=off  Frequencies=[]  VectorFormat=1-D array  Unit=inherit  AffineConversion=off
  Rate Transition1 : RateTransition
  Simulink-PS Converter : nesl_utility/Simulink-PS Converter  PhysicalDomain=network_engine_domain  SubClassName=ps_input  LeftPortType=input  RightPortType=output  PseudoPeriodic=off  Frequencies=[]  NoiseDistribution=none  NoiseParameters=[]  Unit=N*m  AffineConversion=off  FilteringAndDerivatives=provide  SimscapeFilterOrder=1  InputFilterTimeConstant=0.001  UdotUserProvided=0
  "R " : PMIOPort  Side=Right
  MotorSpeed : Outport
  tag scope: theta=global
  wires:
  PS-Simulink Converter1/1 -> [theta]  "angle_motor"
  Gain/1 -> MotorSpeed/1  "speed_motor"
  PS-Simulink Converter/1 -> Gain/1
  Tm/1 -> Data Type Conversion1/1
  Data Type Conversion1/1 -> Gain1/1
  Rate Transition1/1 -> Simulink-PS Converter/1
  Gain1/1 -> Rate Transition1/1
  connections:
  Mechanical Rotational Reference2/LConn1 -- Ideal Rotational Motion Sensor/RConn1
  PS-Simulink Converter1/LConn1 -- Ideal Rotational Motion Sensor/RConn3
  Ideal Rotational Motion Sensor/RConn2 -- PS-Simulink Converter/LConn1
  "R "/RConn1 -- Ideal Rotational Motion Sensor/LConn1 -- Ideal Torque Source/LConn1
  Simulink-PS Converter/RConn1 -- Ideal Torque Source/RConn1
  Mechanical Rotational Reference1/LConn1 -- Ideal Torque Source/RConn2

== system FOC_Motor_Sensorless/FOC Motor/Motor_And_Load/Plant /Simscape/measVI ==
  Current Sensor (Three-Phase) : ee_lib/Sensors & Transducers/Current Sensor (Three-Phase)
  Line Voltage Sensor (Three-Phase) : ee_lib/Sensors & Transducers/Line Voltage Sensor (Three-Phase)
  Low-Pass Filter (Discrete or Continuous) : eeGeneralControl/Low-Pass Filter (Discrete or Continuous)  K=1  T=5e-4  B=inf  A=-inf  init_option=Inherited from block input  x0=0  Ts=-1
  PS-Simulink Converter2 : nesl_utility/PS-Simulink Converter  PhysicalDomain=network_engine_domain  SubClassName=ps_output  LeftPortType=input  RightPortType=output  PseudoPeriodic=off  Frequencies=[]  VectorFormat=1-D array  Unit=inherit  AffineConversion=off
  PS-Simulink Converter3 : nesl_utility/PS-Simulink Converter  PhysicalDomain=network_engine_domain  SubClassName=ps_output  LeftPortType=input  RightPortType=output  PseudoPeriodic=off  Frequencies=[]  VectorFormat=1-D array  Unit=inherit  AffineConversion=off
  ~1 : PMIOPort  Side=Left
  ~2 : PMIOPort  Port=2  Side=Right
  tag scope: Iabc=global, V_ab_bc_ca=global
  wires:
  Low-Pass Filter (Discrete or Continuous)/1 -> [V_ab_bc_ca]
  PS-Simulink Converter3/1 -> [Iabc]  "Iabc"
  PS-Simulink Converter2/1 -> Low-Pass Filter (Discrete or Continuous)/1  "Vabc"
  connections:
  Current Sensor (Three-Phase)/LConn1 -- ~1/RConn1 -- Line Voltage Sensor (Three-Phase)/LConn1
  Current Sensor (Three-Phase)/RConn2 -- ~2/RConn1
  PS-Simulink Converter2/LConn1 -- Line Voltage Sensor (Three-Phase)/RConn1
  Current Sensor (Three-Phase)/RConn1 -- PS-Simulink Converter3/LConn1

== system FOC_Motor_Sensorless/FOC Motor/Controller_Algorithm_Local/Algorithm_HDL/FOC_Current_Control/FOC_Current_Control/DQ_Current_Control ==
  note: DQ Current Control
  Reset : Inport
  Q_Command : Inport  Port=2  SampleTime=sampleTime.CurrentControl
  D_Current : Inport  Port=3
  Q_Current : Inport  Port=4
  D_Command : Constant  Value=0  OutDataTypeStr=fixdt(1,16,0)  SampleTime=-1
  D_Control : slpidlib/PID Controller  Controller=PI  Form=Parallel  TimeDomain=Discrete-time  UseExternalTs=off  SampleTime=-1  IntegratorMethod=Forward Euler  FilterMethod=Forward Euler  ControllerParametersSource=external  P=1  I=1  UseKiTs=on  D=0  UseExternalDerivativeSource=off  N=100  UseFilter=on  TunerSelectOption=Transfer Function Based (PID Tuner App)  InitialConditionSource=internal  InitialConditionForIntegrator=0.1*inverter.V_dc/sqrt(3)  InitialConditionForFilter=0  DifferentiatorICPrevScaledInput=0  ExternalReset=level  TrackingMode=off  Kt=1  LimitOutput=on  SatLimitsSource=internal  UpperSaturationLimit=paramCurrentControlSatVoltage  LowerSaturationLimit=-paramCurrentControlSatVoltage  LinearizeAsGain=on  AntiWindupMode=clamping  Kb=1  LimitIntegrator=off  UpperIntegratorSaturationLimit=inf  LowerIntegratorSaturationLimit=-inf  RndMeth=Simplest  POutMin=[]  POutMax=[]  IOutMin=[]  IOutMax=[]  DOutMin=[]  DOutMax=[]  NOutMin=[]  NOutMax=[]  SumOutMin=[]  SumOutMax=[]  SaturationOutDataTypeStr=Inherit: Inherit via back propagation  SaturationOutMin=[]  SaturationOutMax=[]  PParamMin=[]  PParamMax=[]  IParamMin=[]  IParamMax=[]  DParamMin=[]  DParamMax=[]  NParamMin=[]  NParamMax=[]  KbParamMin=[]  KbParamMax=[]  KtParamMin=[]  KtParamMax=[]  KbOutMin=[]  KbOutMax=[]  KtOutMin=[]  KtOutMax=[]  IntegratorOutMin=[]  IntegratorOutMax=[]  FilterOutMin=[]  FilterOutMax=[]  SumI1OutMin=[]  SumI1OutMax=[]  SumI2OutMin=[]  SumI2OutMax=[]  SumI3OutMin=[]  SumI3OutMax=[]  SumI4OutMin=[]  SumI4OutMax=[]  SumDOutMin=[]  SumDOutMax=[]  DifferentiatorOutMin=[]  DifferentiatorOutMax=[]  FilterDiffOutCoefMin=[]  FilterDiffOutCoefMax=[]  ReciprocalOutMin=[]  ReciprocalOutMax=[]  SumDenOutMin=[]  SumDenOutMax=[]  SumNumOutMin=[]  SumNumOutMax=[]  DivideOutMin=[]  DivideOutMax=[]  UdiffTsProdOutMin=[]  UdiffTsProdOutMax=[]  NTsProdOutMin=[]  NTsProdOutMax=[]  UintegralTsProdOutMin=[]  UintegralTsProdOutMax=[]  UngainTsProdOutMin=[]  UngainTsProdOutMax=[]  ClampingZeroOutDataTypeStr=Inherit: Inherit via back propagation  ClampingZeroOutMin=[]  ClampingZeroOutMax=[]  FilterDenConstantOutDataTypeStr=Inherit: Inherit via back propagation  FilterDenConstantOutMin=[]  FilterDenConstantOutMax=[]  PCopyOutDataTypeStr=Inherit: Inherit via back propagation  PCopyOutMin=[]  PCopyOutMax=[]  NCopyOutDataTypeStr=Inherit: Inherit via back propagation  NCopyOutMin=[]  NCopyOutMax=[]  IntegratorContinuousStateAttributes=''  IntegratorStateMustResolveToSignalObject=off  IntegratorRTWStateStorageClass=Auto  FilterContinuousStateAttributes=''  FilterStateMustResolveToSignalObject=off  FilterRTWStateStorageClass=Auto  ParallelPVariant=ExternalParameters  IdealPVariant=Disabled  IVariant=ExternalParameters  DVariant=Disabled  IntegratorVariant=Discrete  SatVariant=Enabled  AWVariant=DiscClampingParallel  PCopyVariant=Disabled  TRVariant=Disabled  FdbkBlocksVariant=Forward  IdealPFdbkVariant=Disabled  SatFdbkVariant=Disabled  DerivativeFilterVariant=Disabled  NVariant=Disabled  NCopyVariant=Disabled_SignalSpec  FilterICVariant=Disabled  IntegratorICVariant=InternalICs  ExternalResetVariant=ExternalReset  TRSumVariant=Passthrough  SumFdbkVariant=Disabled  SumVariant=Sum_PI  TsampFilterVariant=InternalTs  TsampNgainVariant=Passthrough  TsampIntegralVariant=Disabled_SignalSpec  ExternalSaturationOutDataTypeStr=Inherit: Same as second input  DerivativeSourceVariant=Disabled  PreIntVariant=InternalPreInt
      settings: LibrarySourceBlock=mcblib/Controls/Controllers/PI Controller
  Data_Type_Convert : DataTypeConversion  OutDataTypeStr=fixdt(1,16,11)  RndMeth=Simplest  SaturateOnIntegerOverflow=off
  Data_Type_Convert1 : DataTypeConversion  OutDataTypeStr=fixdt(1,16,11)  RndMeth=Simplest  SaturateOnIntegerOverflow=off
  Error : Sum  Inputs=+-  OutDataTypeStr=fixdt(1,32,24)
  Error1 : Sum  Inputs=+-  OutDataTypeStr=fixdt(1,32,24)
  Integral_Gain : Constant  Value=PI_params.Ki_i  OutDataTypeStr=fixdt(1,16,3)  SampleTime=-1
  Integral_Gain1 : Constant  Value=PI_params.Kp_i  OutDataTypeStr=fixdt(1,16,3)  SampleTime=-1
  Product : Product  OutDataTypeStr=fixdt(1,16,15)
  Q_Control : slpidlib/PID Controller  Controller=PI  Form=Parallel  TimeDomain=Discrete-time  UseExternalTs=off  SampleTime=-1  IntegratorMethod=Forward Euler  FilterMethod=Forward Euler  ControllerParametersSource=external  P=1  I=1  UseKiTs=on  D=0  UseExternalDerivativeSource=off  N=100  UseFilter=on  TunerSelectOption=Transfer Function Based (PID Tuner App)  InitialConditionSource=internal  InitialConditionForIntegrator=0  InitialConditionForFilter=0  DifferentiatorICPrevScaledInput=0  ExternalReset=level  TrackingMode=off  Kt=1  LimitOutput=on  SatLimitsSource=internal  UpperSaturationLimit=paramCurrentControlSatVoltage  LowerSaturationLimit=-paramCurrentControlSatVoltage  LinearizeAsGain=on  AntiWindupMode=clamping  Kb=1  LimitIntegrator=off  UpperIntegratorSaturationLimit=inf  LowerIntegratorSaturationLimit=-inf  RndMeth=Simplest  POutMin=[]  POutMax=[]  IOutMin=[]  IOutMax=[]  DOutMin=[]  DOutMax=[]  NOutMin=[]  NOutMax=[]  SumOutMin=[]  SumOutMax=[]  SaturationOutDataTypeStr=Inherit: Inherit via back propagation  SaturationOutMin=[]  SaturationOutMax=[]  PParamMin=[]  PParamMax=[]  IParamMin=[]  IParamMax=[]  DParamMin=[]  DParamMax=[]  NParamMin=[]  NParamMax=[]  KbParamMin=[]  KbParamMax=[]  KtParamMin=[]  KtParamMax=[]  KbOutMin=[]  KbOutMax=[]  KtOutMin=[]  KtOutMax=[]  IntegratorOutMin=[]  IntegratorOutMax=[]  FilterOutMin=[]  FilterOutMax=[]  SumI1OutMin=[]  SumI1OutMax=[]  SumI2OutMin=[]  SumI2OutMax=[]  SumI3OutMin=[]  SumI3OutMax=[]  SumI4OutMin=[]  SumI4OutMax=[]  SumDOutMin=[]  SumDOutMax=[]  DifferentiatorOutMin=[]  DifferentiatorOutMax=[]  FilterDiffOutCoefMin=[]  FilterDiffOutCoefMax=[]  ReciprocalOutMin=[]  ReciprocalOutMax=[]  SumDenOutMin=[]  SumDenOutMax=[]  SumNumOutMin=[]  SumNumOutMax=[]  DivideOutMin=[]  DivideOutMax=[]  UdiffTsProdOutMin=[]  UdiffTsProdOutMax=[]  NTsProdOutMin=[]  NTsProdOutMax=[]  UintegralTsProdOutMin=[]  UintegralTsProdOutMax=[]  UngainTsProdOutMin=[]  UngainTsProdOutMax=[]  ClampingZeroOutDataTypeStr=Inherit: Inherit via back propagation  ClampingZeroOutMin=[]  ClampingZeroOutMax=[]  FilterDenConstantOutDataTypeStr=Inherit: Inherit via back propagation  FilterDenConstantOutMin=[]  FilterDenConstantOutMax=[]  PCopyOutDataTypeStr=Inherit: Inherit via back propagation  PCopyOutMin=[]  PCopyOutMax=[]  NCopyOutDataTypeStr=Inherit: Inherit via back propagation  NCopyOutMin=[]  NCopyOutMax=[]  IntegratorContinuousStateAttributes=''  IntegratorStateMustResolveToSignalObject=off  IntegratorRTWStateStorageClass=Auto  FilterContinuousStateAttributes=''  FilterStateMustResolveToSignalObject=off  FilterRTWStateStorageClass=Auto  ParallelPVariant=ExternalParameters  IdealPVariant=Disabled  IVariant=ExternalParameters  DVariant=Disabled  IntegratorVariant=Discrete  SatVariant=Enabled  AWVariant=DiscClampingParallel  PCopyVariant=Disabled  TRVariant=Disabled  FdbkBlocksVariant=Forward  IdealPFdbkVariant=Disabled  SatFdbkVariant=Disabled  DerivativeFilterVariant=Disabled  NVariant=Disabled  NCopyVariant=Disabled_SignalSpec  FilterICVariant=Disabled  IntegratorICVariant=InternalICs  ExternalResetVariant=ExternalReset  TRSumVariant=Passthrough  SumFdbkVariant=Disabled  SumVariant=Sum_PI  TsampFilterVariant=InternalTs  TsampNgainVariant=Passthrough  TsampIntegralVariant=Disabled_SignalSpec  ExternalSaturationOutDataTypeStr=Inherit: Same as second input  DerivativeSourceVariant=Disabled  PreIntVariant=InternalPreInt
      settings: LibrarySourceBlock=mcblib/Controls/Controllers/PI Controller
  Reset1 : InportShadow
  Sample_Time : Constant  Value=sampleTime.CurrentControl  OutDataTypeStr=fixdt(1,16,27)  SampleTime=-1
  D_Voltage : Outport  VectorParamsAs1DForOutWhenUnconnected=off
  Q_Voltage : Outport  Port=2  VectorParamsAs1DForOutWhenUnconnected=off
  wires:
  Data_Type_Convert1/1 -> Q_Voltage/1
  D_Control/1 -> Data_Type_Convert/1
  D_Command/1 -> Error/1  "Id_Ref"
  Q_Command/1 -> Error1/1  "Iq_Ref"
  Q_Current/1 -> Error1/2  "Iq_Fb"
  D_Current/1 -> Error/2  "Id_Fb"
  Reset/1 -> D_Control/4
  Reset1/1 -> Q_Control/4
  Error/1 -> D_Control/1  "currentControlError"
  Product/1 -> Q_Control/3, D_Control/3
  Sample_Time/1 -> Product/2
  Integral_Gain/1 -> Product/1
  Integral_Gain1/1 -> Q_Control/2, D_Control/2
  Data_Type_Convert/1 -> D_Voltage/1
  Q_Control/1 -> Data_Type_Convert1/1
  Error1/1 -> Q_Control/1  "currentControlError"

== system FOC_Motor_Sensorless/FOC Motor/Controller_Algorithm_Local/Algorithm_HDL/FOC_Current_Control/FOC_Current_Control/Sine_Cosine ==
  note: Sine Cosine Fixed Point LUT
  P : Inport
  Normalize_Position : Gain  Gain=1/(2*pi)  ParamDataTypeStr=fixdt(1,16,17)  OutMin=0  OutMax=1  OutDataTypeStr=fixdt(1,32,30)
      settings: AttributesFormatString=|
      | ------------------------------
      | Gain = %<Gain>
  Sine_Cosine_LUT : simulink/Lookup Tables/Sine  Formula=sin(2*pi*u) and cos(2*pi*u)  NumDataPoints=(2^5)+1  OutputWordLength=16  InternalRulePriority=Speed
  Sin : Outport  VectorParamsAs1DForOutWhenUnconnected=off
  Cos : Outport  Port=2  VectorParamsAs1DForOutWhenUnconnected=off
  wires:
  Sine_Cosine_LUT/2 -> Cos/1
  Sine_Cosine_LUT/1 -> Sin/1
  Normalize_Position/1 -> Sine_Cosine_LUT/1
  P/1 -> Normalize_Position/1  "position"

== stateflow chart FOC_Motor_Sensorless/FOC Motor/Controller_Algorithm_Local/Algotithm_C/Mode_Scheduler ==
  settings: updateMethod=DISCRETE
  note: Mode Scheduler
  state Enable_Inverter
    state Open_Loop
    state Closed_Loop
    (junction 378) -> Open_Loop [order 1] : [commandType ==  commandTypeEnum.Velocity ]
    (junction 378) -> (junction 627) [order 2]
    Closed_Loop -> Open_Loop [order 2] : [SpeedRef<single(60)]
    Open_Loop -> Closed_Loop : [ SpeedRef >=single(60)]
    Closed_Loop -> (junction 627) [order 1] : [commandType ~= ...
        |  commandTypeEnum.Velocity]
  state Stand_By
    entry:
    if ~adcCalibrationStatus
    adcCalibration = boolean(1);
    end
    exit:
    adcCalibration = boolean(0);
  state Error
  (default) -> Stand_By
  Stand_By -> (junction 378) : [motorOn && adcCalibrationStatus]
  Enable_Inverter -> Stand_By [order 1] : [~motorOn]
  Error -> Stand_By : [~motorOn]
  Enable_Inverter -> Error [order 2] : [error]
  (junction 627) -> Error
  data: mode output Enum: modeSchedulerEnum; enableInverter output boolean; Open_Loop output boolean; motorOn input; commandType input; closedLoop output boolean; SpeedRef input; error input; adcCalibrationStatus input; adcCalibration output

== matlab function FOC_Motor_Sensorless/FOC Motor/Controller_Algorithm_Local/Algotithm_C/ADC_Calibration/MATLAB Function ==
  data: ADCCounts input; ADCOffsetPhA output; Samples input; ADCOffsetPhB output; Flag output; EnCalibration input; ADCOffsets input
function [ADCOffsetPhA, ADCOffsetPhB, Flag]  = fcn(ADCCounts, Samples, EnCalibration, ADCOffsets)

persistent count;
if isempty(count)
	count = single(0);
end

persistent accumulator1;
if isempty(accumulator1) 
	accumulator1 = single(0);
end

persistent accumulator2;
if isempty(accumulator2)
	accumulator2 = single(0);
end
persistent out1; % initalize to meaningful ADC Offset
if isempty(out1)
	out1 = single(ADCOffsets(1));
end
persistent out2;
if isempty(out2)
	out2 = single(ADCOffsets(2));
end
persistent out3;
if isempty(out3)
	out3 = boolean(0);
end

%%
if EnCalibration  % Run the calibration
    if count < Samples
        accumulator1 = accumulator1 + ADCCounts(1);
        accumulator2 = accumulator2 + ADCCounts(2);
        count = count +single(1);
    else
        out1 = single(accumulator1/count);
        out2 = single(accumulator2/count);
        out3 = boolean(1);
    end
    
    ADCOffsetPhA = out1;
    ADCOffsetPhB = out2;
    Flag  = out3; 
else % use the ADC offsets provided 
    ADCOffsetPhA = ADCOffsets(1);
    ADCOffsetPhB = ADCOffsets(2) ;
    Flag  = boolean(1);
end


end

== stateflow chart FOC_Motor_Sensorless/FOC Motor/Controller_Algorithm_Local/Algorithm_HDL/FOC_Current_Control/Over_Current_Detector/Detect_Over_Current_Error ==
  settings: executeAtInitialization=1
  note: Detect Over Current Error
  note: If either Phase A Current (current[0]) or Phase B Current are above the threshold for a given duration, generate an error.
      | The error is reset when over current detection is disabled.
  state No_Error
    entry: error = false;
  state Possible_Error
  state Wait_For_Reset
  state Error
    entry: error = true;
  (default) -> No_Error
  No_Error -> Possible_Error : [enableOverCurrentDetect && ...
      |  ((phaseCurrentA >= overCurrentLimit) || ...
      |   (phaseCurrentB >= overCurrentLimit)    ) ]
  Possible_Error -> No_Error [order 1] : [(phaseCurrentA < overCurrentLimit) && ...
      |  (phaseCurrentB< overCurrentLimit)]
  Wait_For_Reset -> No_Error : [enableOverCurrentDetect]
  Possible_Error -> Error [order 2] : [after(overCurrentDurationTicks,tick)]
  Error -> Wait_For_Reset : [~enableOverCurrentDetect]
  data: enableOverCurrentDetect input; phaseCurrentA input; phaseCurrentB input; overCurrentLimit input; overCurrentDurationTicks input; error output boolean
